simulink model "lab_7_task_4_simulink"  (R2025b)
settings: Solver=ode4  StartTime=0.0  StopTime=100.0  FixedStep=0.01  RelTol=1e-3
values from neighbouring files (symbols this model uses):
  a = 7093    [lab_7_task_1.m]    (also in lab_7_task_2.m; lab_7_task_3.m; lab_7_task_4.m; project_review.m)
  e = 0.5    [lab_7_task_1.m]    (also in lab_7_task_2.m; lab_7_task_3.m = 0.00277; lab_7_task_4.m = 0.00277; project_review.m = 0.00277)
  inc = deg2rad(98.27)    [lab_7_task_1.m]    (also in lab_7_task_2.m; lab_7_task_3.m; lab_7_task_4.m; project_review.m = deg2rad(20))
  n = sqrt(G*M_e/R^3)    [lab_6_task_1.m]    (also in lab_6_task_2.m; lab_7_task_1.m = sqrt(mu_E/(a^3)); lab_7_task_2.m = sqrt(mu_E/(a^3)); lab_7_task_3.m = sqrt(mu/(a^3)))
  TA0 = deg2rad(0)    [lab_7_task_1.m]    (also in lab_7_task_2.m; lab_7_task_3.m; lab_7_task_4.m; project_review.m)
libraries: perturbations x3, dynamics x1, kinematics x1
settings Model: Creator=nicol  LastModifiedBy=nicol

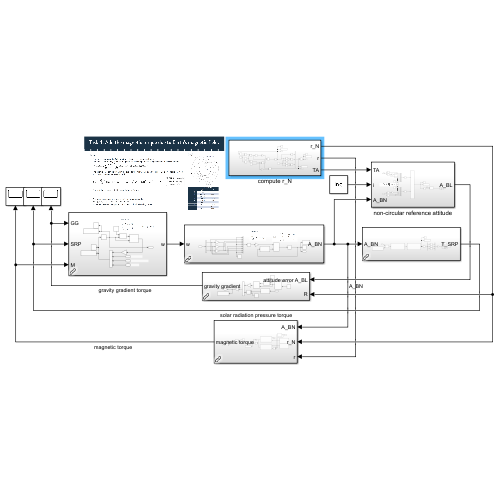
[thumbnail: Simulink's stored preview of the top-level diagram]
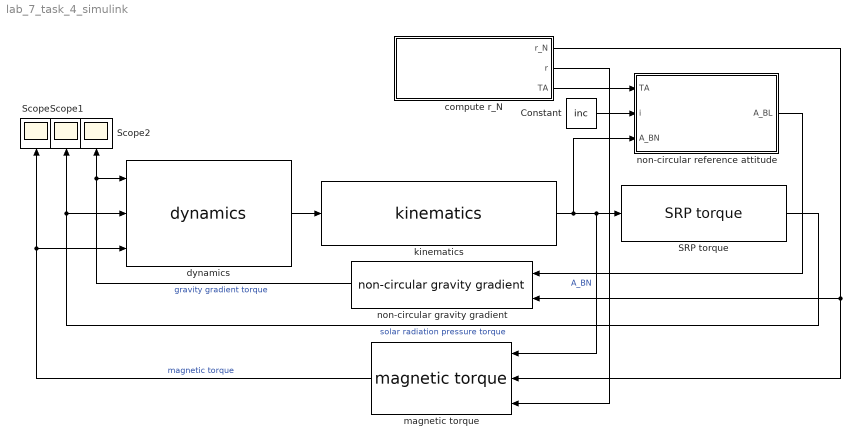
== system lab_7_task_4_simulink ==
  Constant : Constant  Value=inc
  SRP torque : perturbations/SRP torque  SystemSampleTime=-1  VariantActivationTime=update diagram  EmptyChoice=off  PassThrough=off  PassThroughVariantControl=(default)  EmptyChoiceVariantControl=(default)  AllowFlexibleInterface=on  Latency=0  AutoFrameSizeCalculation=off
  Scope : Scope
      settings: ActiveDisplayYMinimum=-1  ActiveDisplayYMaximum=1
  Scope1 : Scope
      settings: ActiveDisplayYMinimum=-3.6448093411352152E-7  ActiveDisplayYMaximum=4.9194799230031577E-7
  Scope2 : Scope
      settings: ActiveDisplayYMinimum=-1  ActiveDisplayYMaximum=1  DataLoggingVariableName=ScopeData4
  compute r_N : Subsystem
  dynamics : dynamics/dynamics  SystemSampleTime=-1  VariantActivationTime=update diagram  EmptyChoice=off  PassThrough=off  PassThroughVariantControl=(default)  EmptyChoiceVariantControl=(default)  AllowFlexibleInterface=on  Latency=0  AutoFrameSizeCalculation=off
  kinematics : kinematics/kinematics  SystemSampleTime=-1  VariantActivationTime=update diagram  EmptyChoice=off  PassThrough=off  PassThroughVariantControl=(default)  EmptyChoiceVariantControl=(default)  AllowFlexibleInterface=on  Latency=0  AutoFrameSizeCalculation=off
  magnetic torque : perturbations/magnetic torque  SystemSampleTime=-1  VariantActivationTime=update diagram  EmptyChoice=off  PassThrough=off  PassThroughVariantControl=(default)  EmptyChoiceVariantControl=(default)  AllowFlexibleInterface=on  Latency=0  AutoFrameSizeCalculation=off
  non-circular gravity gradient : perturbations/non-circular gravity gradient  SystemSampleTime=-1  VariantActivationTime=update diagram  EmptyChoice=off  PassThrough=off  PassThroughVariantControl=(default)  EmptyChoiceVariantControl=(default)  AllowFlexibleInterface=on  Latency=0  AutoFrameSizeCalculation=off
      settings: PortSchema="{\"entries\":[{\"content\":{\"sides\":[{\"content\":{\"connectorIds\":[\"Out1\"]},\"type\":\"ConnectorPlacement.EquallySpacedRectSide\",\"uuid\":\"2a67419a-68c9-4369-a698-e6ac26417455\"},{\"content\":{\"connectorIds\":[\"In1\",\"In2\"],\"side\":\"RIGHT\"},\"type\":\"ConnectorPlacement.EquallySpacedRectSide\",\"uuid\":\"5f3f4c4a-6b79-4b92-8f4c-19ffa36753b2\"},{\"content\":{\"side\":\"TOP\"},\"type\":\"ConnectorPlacement.EquallySpacedRectSide\",\"uuid\":\"22c946b7-ea77-4444-a63c-d5b3d585f671\"}]},\"type\":\"ConnectorPlacement.EquallySpacedConnector\",\"uuid\":\"037c4a72-b28b-418e-a921-9da68dc0cd93\"}],\"packageUris\":[\"http://schema.mathworks.com/mf0/Connector/R2020b\"],\"version\":\"1.0\"}"
  non-circular reference attitude : Subsystem
  wires:
  non-circular gravity gradient/1 -> Scope2/1, dynamics/1  "gravity gradient torque"
  kinematics/1 -> SRP torque/1, magnetic torque/1, non-circular reference attitude/3(A_BN)  "A_BN"
  compute r_N/1(r_N) -> magnetic torque/2, non-circular gravity gradient/2
  compute r_N/3(TA) -> non-circular reference attitude/1(TA)
  Constant/1 -> non-circular reference attitude/2(i)
  dynamics/1 -> kinematics/1
  non-circular reference attitude/1(A_BL) -> non-circular gravity gradient/1
  magnetic torque/1 -> dynamics/3, Scope/1  "magnetic torque"
  SRP torque/1 -> dynamics/2, Scope1/1  "solar radiation pressure torque"
  compute r_N/2(r) -> magnetic torque/3

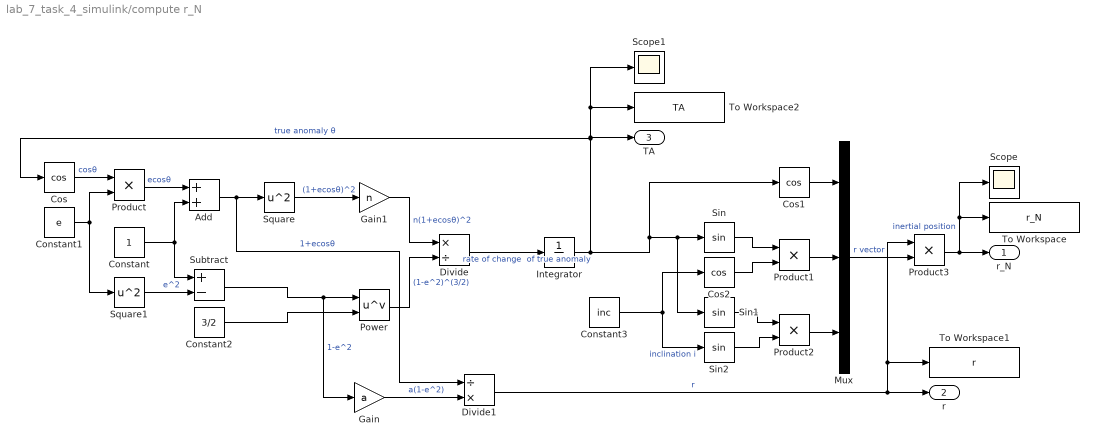
== system lab_7_task_4_simulink/compute r_N ==
  Add : Sum
  Constant : Constant
  Constant1 : Constant  Value=e
  Constant2 : Constant  Value=3/2
  Constant3 : Constant  Value=inc
  Cos : Trigonometry  Operator=cos
  Cos1 : Trigonometry  Operator=cos
  Cos2 : Trigonometry  Operator=cos
  Divide : Product  Inputs=*/
  Divide1 : Product  Inputs=/*
  Gain : Gain  Gain=a
  Gain1 : Gain  Gain=n
  Integrator : Integrator  InitialCondition=TA0
  Mux : Mux  Inputs=3
  Power : Math  Operator=pow
  Product{,1..3} (4 alike) : Product
  Scope : Scope
      settings: ActiveDisplayYMinimum=-1  ActiveDisplayYMaximum=1  DataLoggingVariableName=ScopeData3
  Scope1 : Scope
      settings: ActiveDisplayYMinimum=-1  ActiveDisplayYMaximum=1  DataLoggingVariableName=ScopeData5
  Sin : Trigonometry
  Sin1 : Trigonometry
  Sin2 : Trigonometry
  Square : Math  Operator=square
  Square1 : Math  Operator=square
  Subtract : Sum  Inputs=+-
  To Workspace : ToWorkspace  VariableName=r_N  SaveFormat=Timeseries  SampleTime=-1
  To Workspace1 : ToWorkspace  VariableName=r  SaveFormat=Timeseries  SampleTime=-1
  To Workspace2 : ToWorkspace  VariableName=TA  SaveFormat=Timeseries  SampleTime=-1
  r_N : Outport
  r : Outport  Port=2
  TA : Outport  Port=3
  wires:
  Integrator/1 -> Sin1/1, Sin/1, Cos1/1, TA/1, Scope1/1, To Workspace2/1, Cos/1  "true anomaly θ"
  Add/1 -> Divide1/1, Square/1  "1+ecosθ"
  Square/1 -> Gain1/1  "(1+ecosθ)^2"
  Gain1/1 -> Divide/1  "n(1+ecosθ)^2"
  Sin1/1 -> Product2/1
  Constant/1 -> Subtract/1, Add/2
  Subtract/1 -> Gain/1, Power/1  "1-e^2"
  Product3/1 -> r_N/1, To Workspace/1, Scope/1  "inertial position"
  Constant3/1 -> Cos2/1, Sin2/1  "inclination i"
  Gain/1 -> Divide1/2  "a(1-e^2)"
  Constant2/1 -> Power/2
  Sin2/1 -> Product2/2
  Cos/1 -> Product/1  "cosθ"
  Constant1/1 -> Square1/1, Product/2
  Product/1 -> Add/1  "ecosθ"
  Product2/1 -> Mux/3
  Square1/1 -> Subtract/2  "e^2"
  Divide1/1 -> Product3/1, To Workspace1/1, r/1  "r"
  Cos1/1 -> Mux/1
  Mux/1 -> Product3/2  "r vector"
  Power/1 -> Divide/2  "(1-e^2)^(3/2)"
  Product1/1 -> Mux/2
  Divide/1 -> Integrator/1  "rate of change  of true anomaly"
  Sin/1 -> Product1/1
  Cos2/1 -> Product1/2

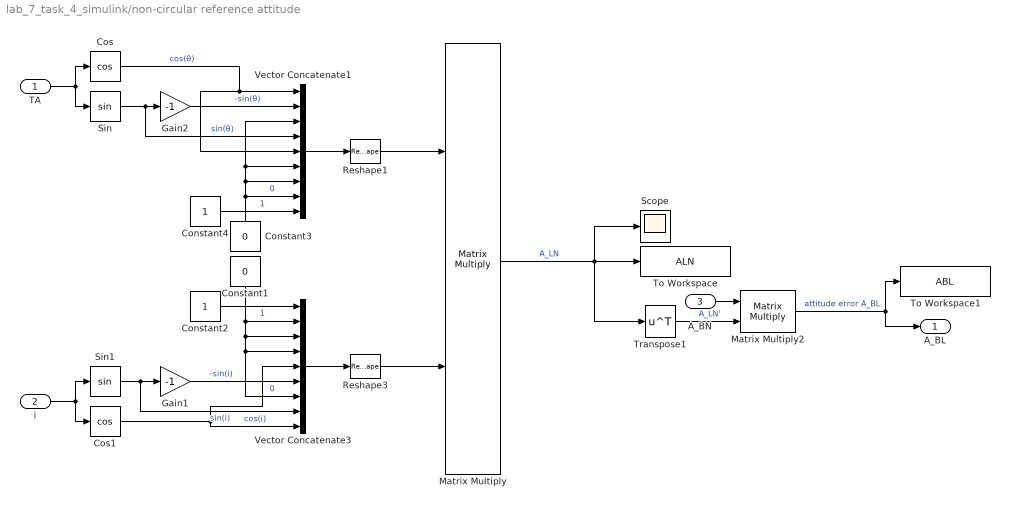
== system lab_7_task_4_simulink/non-circular reference attitude ==
  TA : Inport
  i : Inport  Port=2
  A_BN : Inport  Port=3
  Constant1 : Constant  Value=0
  Constant2 : Constant
  Constant3 : Constant  Value=0
  Constant4 : Constant
  Cos : Trigonometry  Operator=cos
  Cos1 : Trigonometry  Operator=cos
  Gain1 : Gain  Gain=-1
  Gain2 : Gain  Gain=-1
  Matrix Multiply : Product  Multiplication=Matrix(*)
  Matrix Multiply2 : Product  Multiplication=Matrix(*)
  Reshape1 : Reshape  OutputDimensionality=Customize  OutputDimensions=[3,3]
  Reshape3 : Reshape  OutputDimensionality=Customize  OutputDimensions=[3,3]
  Scope : Scope
      settings: ActiveDisplayYMinimum=-1.2499999999912785  ActiveDisplayYMaximum=1.249999999999031  DataLoggingVariableName=ScopeData2
  Sin : Trigonometry
  Sin1 : Trigonometry
  To Workspace : ToWorkspace  VariableName=ALN  SaveFormat=Timeseries  SampleTime=-1
  To Workspace1 : ToWorkspace  VariableName=ABL  SaveFormat=Timeseries  SampleTime=-1
  Transpose1 : Math  Operator=transpose
  Vector Concatenate1 : Concatenate  NumInputs=9
  Vector Concatenate3 : Concatenate  NumInputs=9
  A_BL : Outport
  wires:
  Constant3/1 -> Vector Concatenate1/8, Vector Concatenate1/7, Vector Concatenate1/6, Vector Concatenate1/3  "0"
  TA/1 -> Sin/1, Cos/1
  Gain2/1 -> Vector Concatenate1/2  "-sin(θ)"
  Sin/1 -> Vector Concatenate1/4, Gain2/1  "sin(θ)"
  Matrix Multiply/1 -> Scope/1, Transpose1/1, To Workspace/1  "A_LN"
  Cos/1 -> Vector Concatenate1/5, Vector Concatenate1/1  "cos(θ)"
  Vector Concatenate1/1 -> Reshape1/1
  Constant4/1 -> Vector Concatenate1/9  "1"
  Transpose1/1 -> Matrix Multiply2/2  "A_LN'"
  Reshape1/1 -> Matrix Multiply/1
  Reshape3/1 -> Matrix Multiply/2
  Vector Concatenate3/1 -> Reshape3/1
  Cos1/1 -> Vector Concatenate3/5, Vector Concatenate3/9  "cos(i)"
  Sin1/1 -> Vector Concatenate3/8, Gain1/1  "sin(i)"
  i/1 -> Sin1/1, Cos1/1
  Constant1/1 -> Vector Concatenate3/7, Vector Concatenate3/4, Vector Concatenate3/3, Vector Concatenate3/2  "0"
  Constant2/1 -> Vector Concatenate3/1  "1"
  Gain1/1 -> Vector Concatenate3/6  "-sin(i)"
  A_BN/1 -> Matrix Multiply2/1
  Matrix Multiply2/1 -> To Workspace1/1, A_BL/1  "attitude error A_BL"
